simulink model "OSHW_Multimeter_System"  (R2012b)
settings: Solver=ode45  StartTime=0.0  StopTime=0.005  FixedStep=1/80000000  MaxStep=1/80000000  RelTol=1e-3
undefined symbols (not defined in the file or in its folder): t_pattern, V_th_neg, V_th_pos
settings Model: Creator=Lukas  LastModifiedBy=Lukas

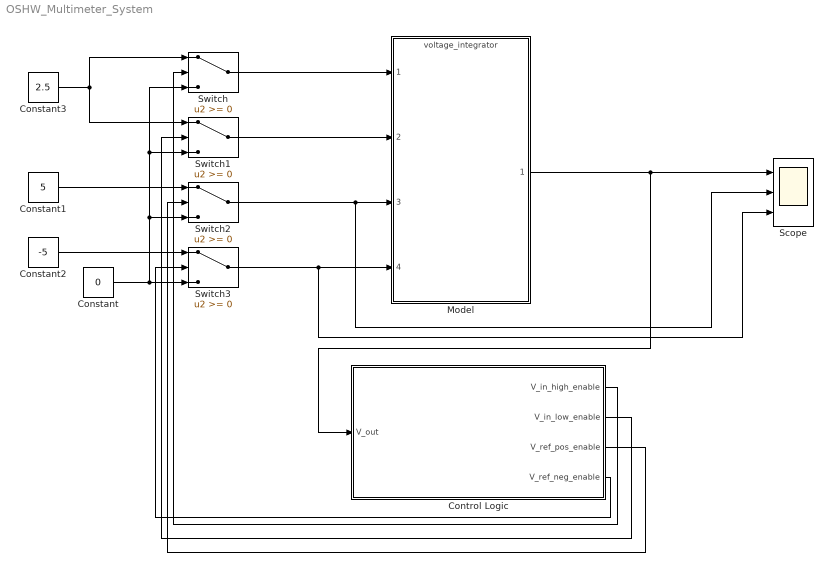
== system OSHW_Multimeter_System ==
  Constant : Constant  Value=0
  Constant1 : Constant  Value=5
  Constant2 : Constant  Value=-5
  Constant3 : Constant  Value=2.5
  Control Logic : Stateflow chart  TreatAsAtomicUnit=on
  Model : ModelReference  ModelNameDialog=voltage_integrator  SimulationMode=Normal  ModelReferenceVersion=1.4  CopyOfModelName=voltage_integrator  DefaultDataLogging=on
  Scope : Scope  NumInputPorts=3
      settings: ShowLegends=on  YMin=-10~0~-5  YMax=10~5~0
  Switch{,1..3} (4 alike) : Switch
  wires:
  Switch1/1 -> Model/2
  Switch2/1 -> Scope/2, Model/3
  Switch3/1 -> Scope/3, Model/4
  Switch/1 -> Model/1
  Constant/1 -> Switch/3, Switch1/3, Switch2/3, Switch3/3
  Constant2/1 -> Switch3/1
  Constant1/1 -> Switch2/1
  Constant3/1 -> Switch/1, Switch1/1
  Model/1 -> Control Logic/1(V_out), Scope/1
  Control Logic/1(V_in_high_enable) -> Switch/2
  Control Logic/2(V_in_low_enable) -> Switch1/2
  Control Logic/3(V_ref_pos_enable) -> Switch2/2
  Control Logic/4(V_ref_neg_enable) -> Switch3/2

== stateflow chart OSHW_Multimeter_System/Control Logic ==
  state Enable_Input
    entry: V_in_high_enable = 1;
    V_in_low_enable = 0;
  state Wait
  state Pattern_1
    state V_neg_on
      en: V_ref_neg_enable = 1;
    state V_pos_on
      en: V_ref_pos_enable = 1;
    state V_neg_off
      en: V_ref_neg_enable = 0;
    state V_pos_off
      en: V_ref_pos_enable = 0;
    Pattern_1.V_neg_on -> Pattern_1.V_pos_on : after(0.35*t_pattern, sec)
    Pattern_1.V_pos_on -> Pattern_1.V_neg_off : after(0.1*t_pattern,sec)
    Pattern_1.V_neg_off -> Pattern_1.V_pos_off : after(0.35*t_pattern,sec)
  state Pattern_4
    state V_pos_on
      en: V_ref_pos_enable = 1;
    state V_neg_on
      en: V_ref_neg_enable = 1;
    state V_neg_off
      en: V_ref_neg_enable = 0;
    state V_pos_off
      en: V_ref_pos_enable = 0;
    Pattern_4.V_pos_on -> Pattern_4.V_neg_on : after(0.35*t_pattern, sec)
    Pattern_4.V_neg_on -> Pattern_4.V_neg_off : after(0.1*t_pattern,sec)
    Pattern_4.V_neg_off -> Pattern_4.V_pos_off : after(0.35*t_pattern,sec)
  state Pattern_3
    state V_neg_on
      en: V_ref_neg_enable = 1;
    state V_pos_on
      en: V_ref_pos_enable = 1;
    state V_pos_off
      en: V_ref_pos_enable = 0;
    state V_neg_off
      en: V_ref_neg_enable = 0;
    Pattern_3.V_neg_on -> Pattern_3.V_pos_on : after(0.35*t_pattern, sec)
    Pattern_3.V_pos_on -> Pattern_3.V_pos_off : after(0.1*t_pattern,sec)
    Pattern_3.V_pos_off -> Pattern_3.V_neg_off : after(0.35*t_pattern,sec)
  state Pattern_2
    state V_pos_on
      en: V_ref_pos_enable = 1;
    state V_neg_on
      en: V_ref_neg_enable = 1;
    state V_pos_off
      en: V_ref_pos_enable = 0;
    state V_neg_off
      en: V_ref_neg_enable = 0;
    Pattern_2.V_pos_on -> Pattern_2.V_neg_on : after(0.35*t_pattern, sec)
    Pattern_2.V_neg_on -> Pattern_2.V_pos_off : after(0.1*t_pattern,sec)
    Pattern_2.V_pos_off -> Pattern_2.V_neg_off : after(0.35*t_pattern,sec)
  (default) -> Enable_Input
  Enable_Input -> Wait
  (junction 76) -> Wait : after(0.1*t_pattern, sec)
  Wait -> (junction 19) : after(0.1*t_pattern, sec)
  (junction 19) -> (junction 31) [order 2] : [V_out < 0 ]
  (junction 19) -> (junction 32) [order 1] : [V_out >= 0 ]
  (junction 31) -> Pattern_1.V_neg_on [order 1] : [V_out > V_th_neg]
  (junction 32) -> Pattern_4.V_pos_on [order 2] : [V_out >= V_th_pos]
  (junction 32) -> Pattern_2.V_pos_on [order 1] : [V_out < V_th_pos]
  (junction 31) -> Pattern_3.V_neg_on [order 2] : [V_out <= V_th_neg]
  Pattern_4.V_pos_off -> (junction 76)
  Pattern_2.V_neg_off -> (junction 76)
  Pattern_1.V_pos_off -> (junction 76)
  Pattern_3.V_neg_off -> (junction 76)
  data: V_out input double size=1; V_in_high_enable output boolean size=1 =0; V_in_low_enable output boolean size=1 =0; V_ref_pos_enable output boolean size=1 =0; V_ref_neg_enable output boolean size=1 =0; V_th_neg parameter; V_th_pos parameter; t_pattern parameter
